simulink model "Cdd_IoHwAb"  (R2024a)
settings: Solver=FixedStepDiscrete  StartTime=0.0  StopTime=10.0  FixedStep=0.01  RelTol=1e-3
settings Model: Creator=gluts  LastModifiedBy=gluts
settings DataIOCC: SaveFormat=StructureWithTime
settings OptimizationCC: DefaultParameterBehavior=Inlined  EnhancedBackFolding=on  PassReuseOutputArgsAs=Individual arguments  ZeroExternalMemoryAtStartup=off  ZeroInternalMemoryAtStartup=off  OptimizeBlockOrder=speed  DifferentSizesBufferReuse=on  OptimizationCustomize=off  EfficientTunableParamExpr=on
settings DebuggingCC: ParameterTunabilityLossMsg=error
settings ModelReferenceCC: ModelReferenceNumInstancesAllowed=Single
settings SFSimCC: MATLABDynamicMemAlloc=off
settings RTWCC: Description=AUTOSAR  SystemTargetFile=autosar.tlc  GenCodeOnly=on  TemplateMakefile=ert_default_tmf  DataTypeReplacement=CDataTypesFixedWidth
settings CodeAppCC: ForceParamTrailComments=on  IgnoreCustomStorageClasses=off  OperatorAnnotations=on  SimulinkDataObjDesc=on  SFDataObjDesc=on  InsertBlockDesc=on
settings STFCustomTargetCC: MultiwordLength=256  ParMdlRefBuildCompliant=on  CompOptLevelCompliant=on  IncludeMdlTerminateFcn=off  CombineOutputUpdateFcns=on  SuppressErrorStatus=on  ERTCustomFileBanners=on  SupportNonFinite=off  SupportComplex=off  SupportContinuousTime=off  SupportNonInlinedSFcns=off  RemoveResetFunc=on  MATLABClassNameForMDSCustomization=Simulink.SoftwareTarget.ERTCustomization  AutosarCompliant=on  GRTInterface=off  LookupTableObjectStructAxisOrder=2,1,3,4,...  LUTObjectStructOrderEvenSpacing=Size,Table,Breakpoints  SystemTargetFile=autosar.tlc
settings ERTTargetCC: TargetLangStandard=C99 (ISO)  ConcurrentExecutionCompliant=off  IncludeMdlTerminateFcn=off  SuppressErrorStatus=on  SupportNonFinite=off  SupportComplex=off  ModelStepFunctionPrototypeControlCompliant=off  CPPClassGenCompliant=off  AutosarCompliant=on  LookupTableObjectStructAxisOrder=2,1,3,4,...  LUTObjectStructOrderEvenSpacing=Size,Table,Breakpoints  InlinedParameterPlacement=NonHierarchical  ERTCustomFileTemplate=example_file_process.tlc  BooleanTrueId=TRUE  BooleanFalseId=FALSE

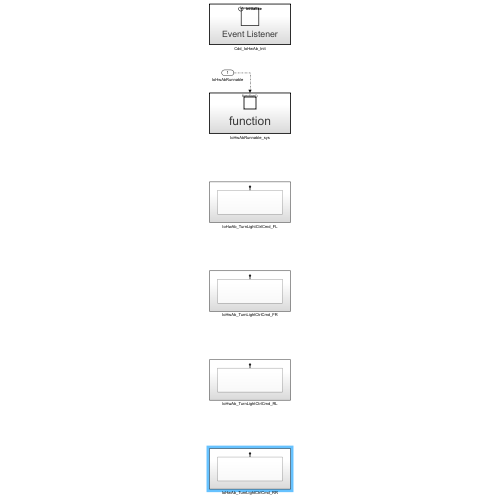
[thumbnail: Simulink's stored preview of the top-level diagram]
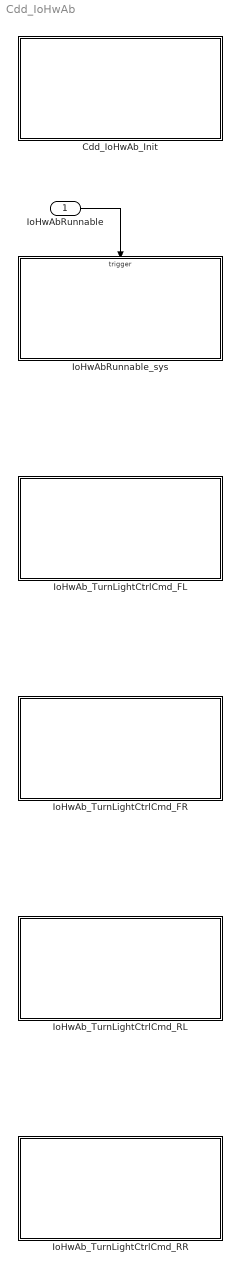
== system Cdd_IoHwAb ==
  IoHwAbRunnable : Inport  SampleTime=0.01  OutputFunctionCall=on
  Cdd_IoHwAb_Init : Subsystem
  IoHwAbRunnable_sys : Subsystem
  IoHwAb_TurnLightCtrlCmd_FL : Subsystem
  IoHwAb_TurnLightCtrlCmd_FR : Subsystem
  IoHwAb_TurnLightCtrlCmd_RL : Subsystem
  IoHwAb_TurnLightCtrlCmd_RR : Subsystem
  wires:
  IoHwAbRunnable/1 -> IoHwAbRunnable_sys/Trigger

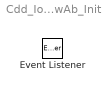
== system Cdd_IoHwAb/Cdd_IoHwAb_Init ==
  Event Listener : EventListener  EventName=reset

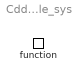
== system Cdd_IoHwAb/IoHwAbRunnable_sys ==
  function : TriggerPort  TriggerType=function-call  VariantControl=(inherit)  SampleTimeType=periodic  SampleTime=-1

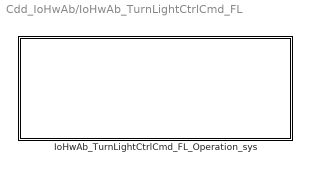
== system Cdd_IoHwAb/IoHwAb_TurnLightCtrlCmd_FL ==
  IoHwAb_TurnLightCtrlCmd_FL_Operation_sys : Subsystem

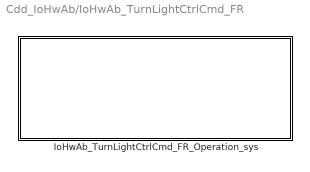
== system Cdd_IoHwAb/IoHwAb_TurnLightCtrlCmd_FR ==
  IoHwAb_TurnLightCtrlCmd_FR_Operation_sys : Subsystem

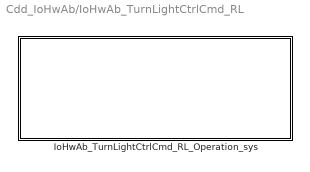
== system Cdd_IoHwAb/IoHwAb_TurnLightCtrlCmd_RL ==
  IoHwAb_TurnLightCtrlCmd_RL_Operation_sys : Subsystem

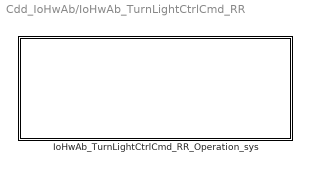
== system Cdd_IoHwAb/IoHwAb_TurnLightCtrlCmd_RR ==
  IoHwAb_TurnLightCtrlCmd_RR_Operation_sys : Subsystem

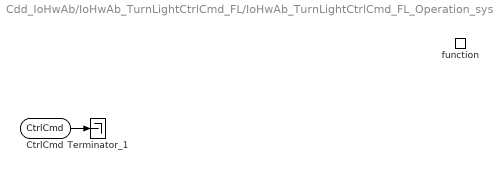
== system Cdd_IoHwAb/IoHwAb_TurnLightCtrlCmd_FL/IoHwAb_TurnLightCtrlCmd_FL_Operation_sys ==
  function : TriggerPort  TriggerType=function-call  IsSimulinkFunction=on  FunctionName=IoHwAb_TurnLightCtrlCmd_FL_Operation  VariantControl=(inherit)
  Terminator_1 : Terminator
  CtrlCmd : ArgIn  OutDataTypeStr=uint8  ArgumentName=CtrlCmd
  wires:
  CtrlCmd/1 -> Terminator_1/1

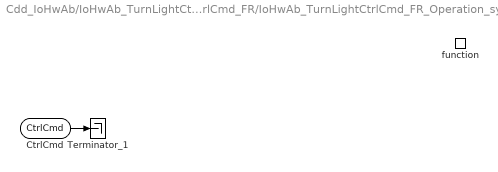
== system Cdd_IoHwAb/IoHwAb_TurnLightCtrlCmd_FR/IoHwAb_TurnLightCtrlCmd_FR_Operation_sys ==
  function : TriggerPort  TriggerType=function-call  IsSimulinkFunction=on  FunctionName=IoHwAb_TurnLightCtrlCmd_FR_Operation  VariantControl=(inherit)
  Terminator_1 : Terminator
  CtrlCmd : ArgIn  OutDataTypeStr=uint8  ArgumentName=CtrlCmd
  wires:
  CtrlCmd/1 -> Terminator_1/1

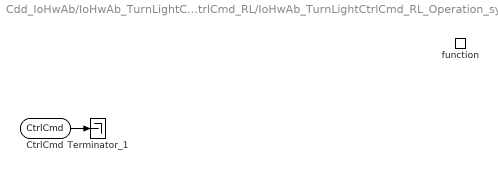
== system Cdd_IoHwAb/IoHwAb_TurnLightCtrlCmd_RL/IoHwAb_TurnLightCtrlCmd_RL_Operation_sys ==
  function : TriggerPort  TriggerType=function-call  IsSimulinkFunction=on  FunctionName=IoHwAb_TurnLightCtrlCmd_RL_Operation  VariantControl=(inherit)
  Terminator_1 : Terminator
  CtrlCmd : ArgIn  OutDataTypeStr=uint8  ArgumentName=CtrlCmd
  wires:
  CtrlCmd/1 -> Terminator_1/1

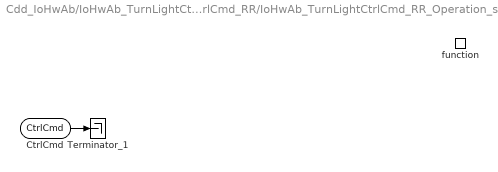
== system Cdd_IoHwAb/IoHwAb_TurnLightCtrlCmd_RR/IoHwAb_TurnLightCtrlCmd_RR_Operation_sys ==
  function : TriggerPort  TriggerType=function-call  IsSimulinkFunction=on  FunctionName=IoHwAb_TurnLightCtrlCmd_RR_Operation  VariantControl=(inherit)
  Terminator_1 : Terminator
  CtrlCmd : ArgIn  OutDataTypeStr=uint8  ArgumentName=CtrlCmd
  wires:
  CtrlCmd/1 -> Terminator_1/1
